simulink model "plainMRAC"  (R2022a)
settings: Solver=VariableStepAuto  StartTime=0.0  StopTime=50  RelTol=1e-3
undefined symbols (not defined in the file): a, a_m, b, b_m, c
settings Model: Creator=edgar  LastModifiedBy=edgar

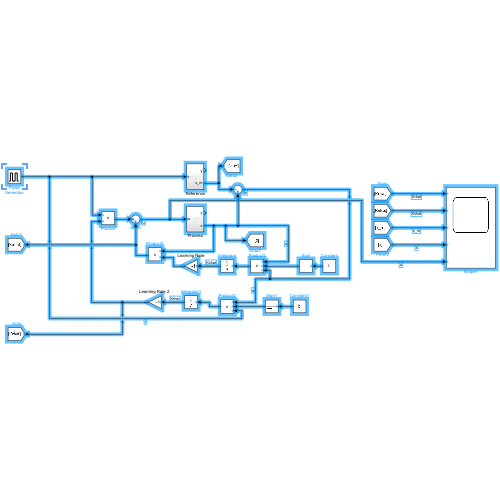
[thumbnail: Simulink's stored preview of the top-level diagram]
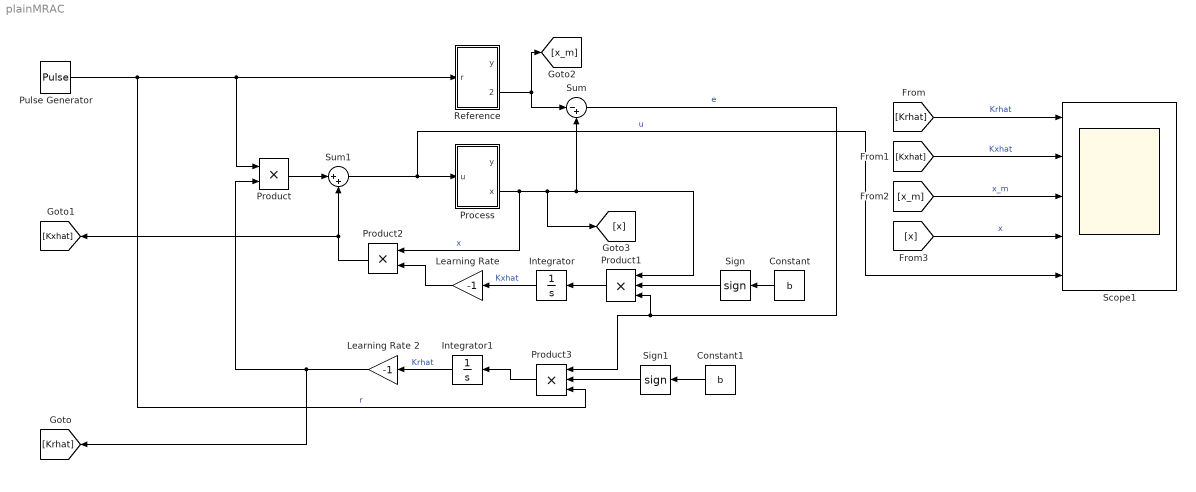
== system plainMRAC ==
  Constant : Constant  Value=b
  Constant1 : Constant  Value=b
  Integrator : Integrator
  Integrator1 : Integrator
  Learning Rate : Gain  Gain=-1
  "Learning Rate 2 " : Gain  Gain=-1
  Process : Subsystem
  Product : Product
  Product1 : Product  Inputs=3
  Product2 : Product
  Product3 : Product  Inputs=3
  Pulse Generator : DiscretePulseGenerator  PulseType=Time based  Amplitude=10  Period=10  PulseWidth=50
  Reference : Subsystem
  Scope1 : Scope  NumInputPorts=5
  Sign : Signum
  Sign1 : Signum
  Sum : Sum  Inputs=|-+
  Sum1 : Sum  Inputs=|++
  wires:
  Constant/1 -> Sign/1
  [Krhat] -> Scope1/1  "Krhat"
  Sign1/1 -> Product3/2
  Product/1 -> Sum1/1
  Pulse Generator/1 -> Product3/3, Reference/1(r), Product/1  "r"
  [x_m] -> Scope1/3  "x_m"
  Integrator1/1 -> "Learning Rate 2 "/1  "Krhat"
  Sum/1 -> Product3/1, Product1/3  "e"
  "Learning Rate 2 "/1 -> [Krhat], Product/2
  Sign/1 -> Product1/2
  [Kxhat] -> Scope1/2  "Kxhat"
  Constant1/1 -> Sign1/1
  Learning Rate/1 -> Product2/2
  Product3/1 -> Integrator1/1
  Sum1/1 -> Scope1/5, Process/1(u)  "u"
  Reference/2(x_m) -> [x_m], Sum/1
  [x] -> Scope1/4  "x"
  Integrator/1 -> Learning Rate/1  "Kxhat"
  Product2/1 -> [Kxhat], Sum1/2
  Product1/1 -> Integrator/1
  Process/2(x) -> Product2/1, [x], Product1/1, Sum/2  "x"

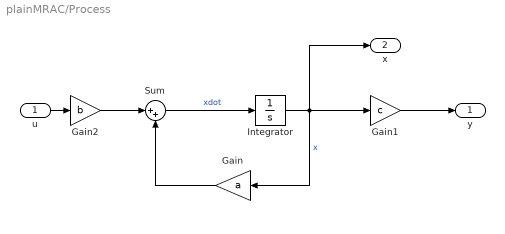
== system plainMRAC/Process ==
  u : Inport
  Gain : Gain  Gain=a
  Gain1 : Gain  Gain=c
  Gain2 : Gain  Gain=b
  Integrator : Integrator
  Sum : Sum  Inputs=|++
  y : Outport
  x : Outport  Port=2
  wires:
  Sum/1 -> Integrator/1  "xdot"
  Integrator/1 -> x/1, Gain1/1, Gain/1  "x"
  Gain1/1 -> y/1
  Gain2/1 -> Sum/1
  Gain/1 -> Sum/2
  u/1 -> Gain2/1

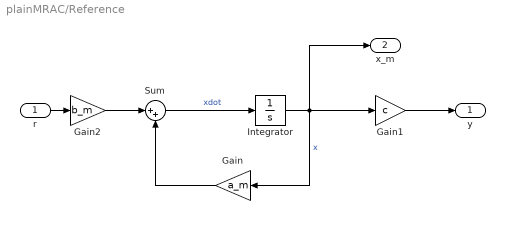
== system plainMRAC/Reference ==
  r : Inport
  Gain : Gain  Gain=a_m
  Gain1 : Gain  Gain=c
  Gain2 : Gain  Gain=b_m
  Integrator : Integrator
  Sum : Sum  Inputs=|++
  y : Outport
  x_m : Outport  Port=2
  wires:
  Sum/1 -> Integrator/1  "xdot"
  Integrator/1 -> x_m/1, Gain1/1, Gain/1  "x"
  Gain1/1 -> y/1
  Gain2/1 -> Sum/1
  Gain/1 -> Sum/2
  r/1 -> Gain2/1
